simulink model "simulazione"  (R2022b)
settings: Solver=VariableStepAuto  StartTime=0.0  StopTime=100  RelTol=1e-3
values from neighbouring files (symbols this model uses):
  Controller = ss(Ctrl)    [runme.m]
  System = ss(G)    [runme.m]
settings Model: Creator=marco  LastModifiedBy=davidebonura
settings SolverCC: AlgebraicLoopSolver=TrustRegion
settings DataIOCC: ReturnWorkspaceOutputs=off
settings DebuggingCC: UnconnectedInputMsg=warning  UnconnectedOutputMsg=warning  UnconnectedLineMsg=warning  SFMachineParentedDataDiag=warning  ArithmeticOperatorsInVariantConditions=warning
settings ModelReferenceCC: EnableRefExpFcnMdlSchedulingChecks=on
settings SFSimCC: CustomCodeUndefinedFunction=UseInterfaceOnly

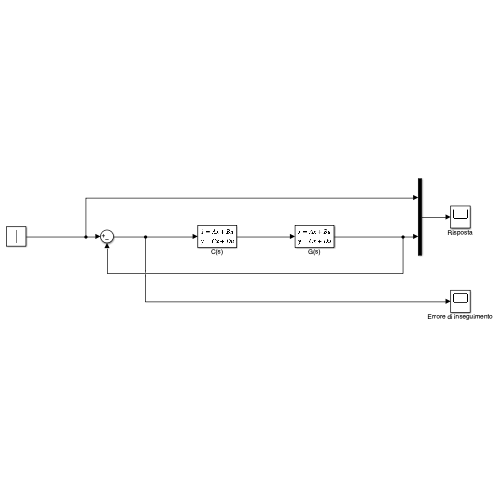
[thumbnail: Simulink's stored preview of the top-level diagram]
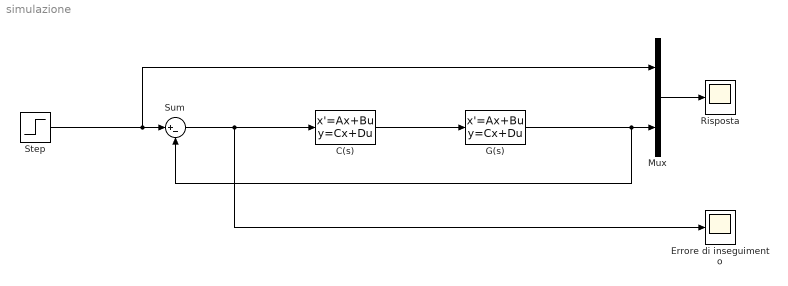
== system simulazione ==
  C(s) : StateSpace  A=Controller.A  B=Controller.B  C=Controller.C  D=Controller.D  InitialCondition=0
  Errore di inseguimento : Scope
  G(s) : StateSpace  A=System.A  B=System.B  C=System.C  D=System.D  InitialCondition=0
  Mux : Mux  Inputs=2
  "Risposta " : Scope
  Step : Step  Time=0  SampleTime=0
  Sum : Sum  Inputs=|+-
  wires:
  Step/1 -> Mux/1, Sum/1
  Sum/1 -> Errore di inseguimento/1, C(s)/1
  C(s)/1 -> G(s)/1
  Mux/1 -> "Risposta "/1
  G(s)/1 -> Sum/2, Mux/2
